simulink model "robot_uniciclo"  (R2024b)
settings: Solver=VariableStepAuto  StartTime=0.0  StopTime=10.0
settings Model: Creator=Utente  LastModifiedBy=david

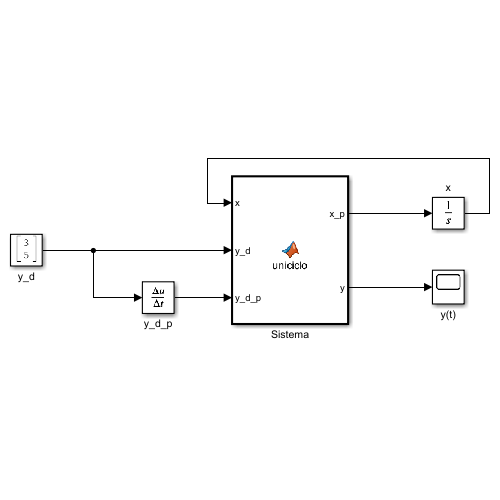
[thumbnail: Simulink's stored preview of the top-level diagram]
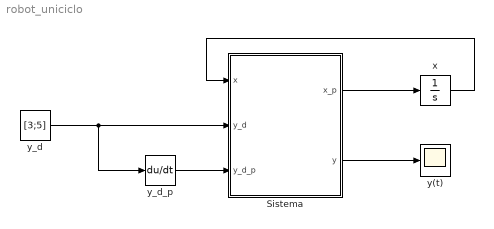
== system robot_uniciclo ==
  Sistema : MATLAB Function  TreatAsAtomicUnit=on
  x : Integrator  InitialCondition=[0;0]  ZeroCross=off
  y(t) : Scope
  y_d : Constant  Value=[3;5]  VectorParams1D=off
  y_d_p : Derivative
  wires:
  y_d/1 -> y_d_p/1, Sistema/2(y_d)
  y_d_p/1 -> Sistema/3(y_d_p)
  Sistema/1(x_p) -> x/1
  Sistema/2(y) -> y(t)/1
  x/1 -> Sistema/1(x)

== matlab function robot_uniciclo/Sistema ==
  data: x_p output; x input; y output; y_d input; y_d_p input
function [x_p,y] = uniciclo(x,y_d,y_d_p)

%Definizione parametri
k1 = 2;
k2 = 2;
b = 0.3;
theta = atan2(y_d(2) - x(2) , y_d(1) - x(1));

%Uscite
y = [x(1) + b*cos(theta);
     x(2) + b*sin(theta)];

%Regolazione
u = y_d_p + [k1,0;0,k2]*(y_d-y);

%Definizione matrice T inversa
T_inv = [ cos(theta),    sin(theta)  ;
         -sin(theta)/b,  cos(theta)/b];

%Calcolo delle velocità
v_w = T_inv*u;
v = v_w(1);

%Calcolo della dinamica 
x_p = [v*cos(theta);
       v*sin(theta)];
